simulink model "npc_controller"  (R2022a)
settings: Solver=FixedStepDiscrete  StartTime=0.0  StopTime=20  RelTol=1e-3  EnableMultiTasking=on
undefined symbols (not defined in the file): CAN_O_INT, CANA_BASE, Down, GPTRIP1SEL, GPTRIP2SEL, GPTRIP3SEL, Tsw, TZ1, TZ2, TZ3, Up, V2G_en
libraries: simulink x171, hdlsllib x90, c2802xlib x46, c2837xDlib x19, c280xlib x12, canmsglib x9, c2838xlib x8, idelinklib_common x5, c2806xlib x2, slpidlib x2, c28004xlib x2, c281xlib x2
(part 49 of 55)

== system npc_controller/CONTROL/STATE-MACHINE/CPU_CONTROL_100_A2_precharge_pfc_ok2/configGrid/FORCE_TZ/1P/LEG_A/System Outputs2 ==

== system npc_controller/CONTROL/STATE-MACHINE/CPU_CONTROL_100_A2_precharge_pfc_ok2/configGrid/FORCE_TZ/1P/LEG_B/System Outputs2 ==

== system npc_controller/CONTROL/STATE-MACHINE/CPU_CONTROL_100_A2_precharge_pfc_ok2/configGrid/FORCE_TZ/1P/LEG_C/System Outputs2 ==

== system npc_controller/CONTROL/STATE-MACHINE/CPU_CONTROL_100_A2_precharge_pfc_ok2/updatePll3p/PLL/SRF_PLL/Integrator/Accumulation ==
  In1 : Inport  OutDataTypeStr=single
  Action Port : ActionPort
  Out : Outport  OutDataTypeStr=single
  wires:
  In1/1 -> Out/1

== system npc_controller/CONTROL/STATE-MACHINE/CPU_CONTROL_100_A2_precharge_pfc_ok2/updatePll3p/PLL/SRF_PLL/Integrator/Reset Integrator ==
  Action Port : ActionPort
  Constant1 : Constant  Value=0  OutDataTypeStr=single
  Out : Outport
  wires:
  Constant1/1 -> Out/1

== system npc_controller/CONTROL/STATE-MACHINE/CPU_CONTROL_100_inv/configGrid/FORCE_TZ/1P/ALL_LEGS/System Outputs2 ==

== system npc_controller/CONTROL/STATE-MACHINE/CPU_CONTROL_100_inv/configGrid/FORCE_TZ/1P/LEG_A/System Outputs2 ==

== system npc_controller/CONTROL/STATE-MACHINE/CPU_CONTROL_100_inv/configGrid/FORCE_TZ/1P/LEG_B/System Outputs2 ==

== system npc_controller/CONTROL/STATE-MACHINE/CPU_CONTROL_100_inv/configGrid/FORCE_TZ/1P/LEG_C/System Outputs2 ==

== system npc_controller/CONTROL/STATE-MACHINE/CPU_CONTROL_100_inv/updatePll3p/PLL/SRF_PLL/Integrator/Accumulation ==
  In1 : Inport  OutDataTypeStr=single
  Action Port : ActionPort
  Out : Outport  OutDataTypeStr=single
  wires:
  In1/1 -> Out/1

== system npc_controller/CONTROL/STATE-MACHINE/CPU_CONTROL_100_inv/updatePll3p/PLL/SRF_PLL/Integrator/Reset Integrator ==
  Action Port : ActionPort
  Constant1 : Constant  Value=0  OutDataTypeStr=single
  Out : Outport
  wires:
  Constant1/1 -> Out/1

== system npc_controller/CONTROL/STATE-MACHINE/CPU_CONTROL_100_inv/updateSequencePhA/pol_vxn1/neg/SR OFF/System Outputs1 ==

== system npc_controller/CONTROL/STATE-MACHINE/CPU_CONTROL_100_inv/updateSequencePhA/pol_vxn1/neg/SR OFF/System Outputs2 ==

== system npc_controller/CONTROL/STATE-MACHINE/CPU_CONTROL_100_inv/updateSequencePhA/pol_vxn1/neg/SR ON/System Outputs1 ==

== system npc_controller/CONTROL/STATE-MACHINE/CPU_CONTROL_100_inv/updateSequencePhA/pol_vxn1/neg/SR ON/System Outputs2 ==

== system npc_controller/CONTROL/STATE-MACHINE/CPU_CONTROL_100_inv/updateSequencePhA/pol_vxn1/neg/SR ON1/System Outputs1 ==

== system npc_controller/CONTROL/STATE-MACHINE/CPU_CONTROL_100_inv/updateSequencePhA/pol_vxn1/neg/SR ON1/System Outputs2 ==

== system npc_controller/CONTROL/STATE-MACHINE/CPU_CONTROL_100_inv/updateSequencePhA/pol_vxn1/pos/S3_Blanking/System Outputs1 ==

== system npc_controller/CONTROL/STATE-MACHINE/CPU_CONTROL_100_inv/updateSequencePhA/pol_vxn1/pos/S3_Blanking/System Outputs2 ==

== system npc_controller/CONTROL/STATE-MACHINE/CPU_CONTROL_100_inv/updateSequencePhA/pol_vxn1/pos/SR Force to Low/System Outputs1 ==

== system npc_controller/CONTROL/STATE-MACHINE/CPU_CONTROL_100_inv/updateSequencePhA/pol_vxn1/pos/SR Force to Low/System Outputs2 ==

== system npc_controller/CONTROL/STATE-MACHINE/CPU_CONTROL_100_inv/updateSequencePhA/pol_vxn1/pos/SR ON/System Outputs1 ==

== system npc_controller/CONTROL/STATE-MACHINE/CPU_CONTROL_100_inv/updateSequencePhA/pol_vxn1/pos/SR ON/System Outputs2 ==

== system npc_controller/CONTROL/STATE-MACHINE/CPU_CONTROL_100_inv/updateSequencePhA1/pol_vxn1/neg/SR OFF/System Outputs1 ==

== system npc_controller/CONTROL/STATE-MACHINE/CPU_CONTROL_100_inv/updateSequencePhA1/pol_vxn1/neg/SR OFF/System Outputs2 ==

== system npc_controller/CONTROL/STATE-MACHINE/CPU_CONTROL_100_inv/updateSequencePhA1/pol_vxn1/neg/SR ON/System Outputs1 ==

== system npc_controller/CONTROL/STATE-MACHINE/CPU_CONTROL_100_inv/updateSequencePhA1/pol_vxn1/neg/SR ON/System Outputs2 ==

== system npc_controller/CONTROL/STATE-MACHINE/CPU_CONTROL_100_inv/updateSequencePhA1/pol_vxn1/pos/SR Force to Low/System Outputs1 ==

== system npc_controller/CONTROL/STATE-MACHINE/CPU_CONTROL_100_inv/updateSequencePhA1/pol_vxn1/pos/SR Force to Low/System Outputs2 ==

== system npc_controller/CONTROL/STATE-MACHINE/CPU_CONTROL_100_inv/updateSequencePhA1/pol_vxn1/pos/SR ON/System Outputs1 ==

== system npc_controller/CONTROL/STATE-MACHINE/CPU_CONTROL_100_inv/updateSequencePhA1/pol_vxn1/pos/SR ON/System Outputs2 ==

== system npc_controller/CONTROL/STATE-MACHINE/CPU_CONTROL_100_inv/updateSequencePhB/pol_vxn1/neg/SR OFF/System Outputs2 ==

== system npc_controller/CONTROL/STATE-MACHINE/CPU_CONTROL_100_inv/updateSequencePhB/pol_vxn1/neg/SR ON/System Outputs1 ==

== system npc_controller/CONTROL/STATE-MACHINE/CPU_CONTROL_100_inv/updateSequencePhB/pol_vxn1/neg/SR ON1/System Outputs1 ==

== system npc_controller/CONTROL/STATE-MACHINE/CPU_CONTROL_100_inv/updateSequencePhB/pol_vxn1/pos/SR Force to Low/System Outputs2 ==

== system npc_controller/CONTROL/STATE-MACHINE/CPU_CONTROL_100_inv/updateSequencePhB/pol_vxn1/pos/SR ON/System Outputs1 ==

== system npc_controller/CONTROL/STATE-MACHINE/CPU_CONTROL_100_inv/updateSequencePhB/pol_vxn1/pos/SR ON1/System Outputs1 ==

== system npc_controller/CONTROL/STATE-MACHINE/CPU_CONTROL_100_inv/updateSequencePhB1/pol_vxn1/neg/SR OFF/System Outputs2 ==

== system npc_controller/CONTROL/STATE-MACHINE/CPU_CONTROL_100_inv/updateSequencePhB1/pol_vxn1/neg/SR ON/System Outputs1 ==

== system npc_controller/CONTROL/STATE-MACHINE/CPU_CONTROL_100_inv/updateSequencePhB1/pol_vxn1/pos/SR Force to Low/System Outputs2 ==

== system npc_controller/CONTROL/STATE-MACHINE/CPU_CONTROL_100_inv/updateSequencePhB1/pol_vxn1/pos/SR ON/System Outputs1 ==

== system npc_controller/CONTROL/STATE-MACHINE/CPU_CONTROL_100_inv/updateSequencePhC/pol_vxn1/neg/S2_Blanking/System Outputs1 ==

== system npc_controller/CONTROL/STATE-MACHINE/CPU_CONTROL_100_inv/updateSequencePhC/pol_vxn1/neg/SR OFF/System Outputs1 ==

== system npc_controller/CONTROL/STATE-MACHINE/CPU_CONTROL_100_inv/updateSequencePhC/pol_vxn1/neg/SR ON/System Outputs1 ==

== system npc_controller/CONTROL/STATE-MACHINE/CPU_CONTROL_100_inv/updateSequencePhC/pol_vxn1/pos/S3_Blanking/System Outputs1 ==

== system npc_controller/CONTROL/STATE-MACHINE/CPU_CONTROL_100_inv/updateSequencePhC/pol_vxn1/pos/SR Force to Low/System Outputs2 ==

== system npc_controller/CONTROL/STATE-MACHINE/CPU_CONTROL_100_inv/updateSequencePhC/pol_vxn1/pos/SR ON/System Outputs1 ==

== system npc_controller/CONTROL/STATE-MACHINE/CPU_CONTROL_100_inv/updateSequencePhC1/pol_vxn1/neg/SR OFF/System Outputs1 ==

== system npc_controller/CONTROL/STATE-MACHINE/CPU_CONTROL_100_inv/updateSequencePhC1/pol_vxn1/neg/SR ON/System Outputs1 ==

== system npc_controller/CONTROL/STATE-MACHINE/CPU_CONTROL_100_inv/updateSequencePhC1/pol_vxn1/pos/SR Force to Low/System Outputs2 ==

== system npc_controller/CONTROL/STATE-MACHINE/CPU_CONTROL_100_inv/updateSequencePhC1/pol_vxn1/pos/SR ON/System Outputs1 ==

== system npc_controller/CONTROL/STATE-MACHINE/CPU_CONTROL_200_A2_precharge_pfc_ok2/configGrid/FORCE_TZ/1P/ALL_LEGS/System Outputs2 ==

== system npc_controller/CONTROL/STATE-MACHINE/CPU_CONTROL_200_A2_precharge_pfc_ok2/configGrid/FORCE_TZ/1P/LEG_A/System Outputs2 ==

== system npc_controller/CONTROL/STATE-MACHINE/CPU_CONTROL_200_A2_precharge_pfc_ok2/configGrid/FORCE_TZ/1P/LEG_B/System Outputs2 ==

== system npc_controller/CONTROL/STATE-MACHINE/CPU_CONTROL_200_A2_precharge_pfc_ok2/configGrid/FORCE_TZ/1P/LEG_C/System Outputs2 ==

== system npc_controller/CONTROL/STATE-MACHINE/CPU_CONTROL_200_A2_precharge_pfc_ok2/updatePll3p/PLL/SRF_PLL/Integrator/Accumulation ==
  In1 : Inport  OutDataTypeStr=single
  Action Port : ActionPort
  Out : Outport  OutDataTypeStr=single
  wires:
  In1/1 -> Out/1

== system npc_controller/CONTROL/STATE-MACHINE/CPU_CONTROL_200_A2_precharge_pfc_ok2/updatePll3p/PLL/SRF_PLL/Integrator/Reset Integrator ==
  Action Port : ActionPort
  Constant1 : Constant  Value=0  OutDataTypeStr=single
  Out : Outport
  wires:
  Constant1/1 -> Out/1

== system npc_controller/CONTROL/STATE-MACHINE/CPU_CONTROL_200_A2_precharge_pfc_ok2_OL SS/configGrid/FORCE_TZ/1P/ALL_LEGS/System Outputs2 ==

== system npc_controller/CONTROL/STATE-MACHINE/CPU_CONTROL_200_A2_precharge_pfc_ok2_OL SS/configGrid/FORCE_TZ/1P/LEG_A/System Outputs2 ==

== system npc_controller/CONTROL/STATE-MACHINE/CPU_CONTROL_200_A2_precharge_pfc_ok2_OL SS/configGrid/FORCE_TZ/1P/LEG_B/System Outputs2 ==

== system npc_controller/CONTROL/STATE-MACHINE/CPU_CONTROL_200_A2_precharge_pfc_ok2_OL SS/configGrid/FORCE_TZ/1P/LEG_C/System Outputs2 ==

== system npc_controller/CONTROL/STATE-MACHINE/CPU_CONTROL_200_A2_precharge_pfc_ok2_OL SS/updatePll3p/PLL/SRF_PLL/Integrator/Accumulation ==
  In1 : Inport  OutDataTypeStr=single
  Action Port : ActionPort
  Out : Outport  OutDataTypeStr=single
  wires:
  In1/1 -> Out/1

== system npc_controller/CONTROL/STATE-MACHINE/CPU_CONTROL_200_A2_precharge_pfc_ok2_OL SS/updatePll3p/PLL/SRF_PLL/Integrator/Reset Integrator ==
  Action Port : ActionPort
  Constant1 : Constant  Value=0  OutDataTypeStr=single
  Out : Outport
  wires:
  Constant1/1 -> Out/1

== system npc_controller/CONTROL/STATE-MACHINE/CPU_CONTROL_200_Vpk/configGrid/FORCE_TZ/1P/ALL_LEGS/System Outputs2 ==

== system npc_controller/CONTROL/STATE-MACHINE/CPU_CONTROL_200_Vpk/configGrid/FORCE_TZ/1P/LEG_A/System Outputs2 ==

== system npc_controller/CONTROL/STATE-MACHINE/CPU_CONTROL_200_Vpk/configGrid/FORCE_TZ/1P/LEG_B/System Outputs2 ==

== system npc_controller/CONTROL/STATE-MACHINE/CPU_CONTROL_200_Vpk/configGrid/FORCE_TZ/1P/LEG_C/System Outputs2 ==

== system npc_controller/CONTROL/STATE-MACHINE/CPU_CONTROL_200_Vpk/updatePll3p/PLL/SRF_PLL/Integrator/Accumulation ==
  In1 : Inport  OutDataTypeStr=single
  Action Port : ActionPort
  Out : Outport  OutDataTypeStr=single
  wires:
  In1/1 -> Out/1

== system npc_controller/CONTROL/STATE-MACHINE/CPU_CONTROL_200_Vpk/updatePll3p/PLL/SRF_PLL/Integrator/Reset Integrator ==
  Action Port : ActionPort
  Constant1 : Constant  Value=0  OutDataTypeStr=single
  Out : Outport
  wires:
  Constant1/1 -> Out/1

== system npc_controller/CONTROL/STATE-MACHINE/CPU_CONTROL_200_inv/configGrid/FORCE_TZ/1P/ALL_LEGS/System Outputs2 ==

== system npc_controller/CONTROL/STATE-MACHINE/CPU_CONTROL_200_inv/configGrid/FORCE_TZ/1P/LEG_A/System Outputs2 ==

== system npc_controller/CONTROL/STATE-MACHINE/CPU_CONTROL_200_inv/configGrid/FORCE_TZ/1P/LEG_B/System Outputs2 ==

== system npc_controller/CONTROL/STATE-MACHINE/CPU_CONTROL_200_inv/configGrid/FORCE_TZ/1P/LEG_C/System Outputs2 ==

== system npc_controller/CONTROL/STATE-MACHINE/CPU_CONTROL_200_inv/updatePll3p/PLL/SRF_PLL/Integrator/Accumulation ==
  In1 : Inport  OutDataTypeStr=single
  Action Port : ActionPort
  Out : Outport  OutDataTypeStr=single
  wires:
  In1/1 -> Out/1

== system npc_controller/CONTROL/STATE-MACHINE/CPU_CONTROL_200_inv/updatePll3p/PLL/SRF_PLL/Integrator/Reset Integrator ==
  Action Port : ActionPort
  Constant1 : Constant  Value=0  OutDataTypeStr=single
  Out : Outport
  wires:
  Constant1/1 -> Out/1

== system npc_controller/CONTROL/STATE-MACHINE/CPU_CONTROL_200_inv/updateSequencePhA/pol_vxn1/neg/SR OFF/System Outputs1 ==

== system npc_controller/CONTROL/STATE-MACHINE/CPU_CONTROL_200_inv/updateSequencePhA/pol_vxn1/neg/SR OFF/System Outputs2 ==

== system npc_controller/CONTROL/STATE-MACHINE/CPU_CONTROL_200_inv/updateSequencePhA/pol_vxn1/neg/SR ON/System Outputs1 ==

== system npc_controller/CONTROL/STATE-MACHINE/CPU_CONTROL_200_inv/updateSequencePhA/pol_vxn1/neg/SR ON/System Outputs2 ==

== system npc_controller/CONTROL/STATE-MACHINE/CPU_CONTROL_200_inv/updateSequencePhA/pol_vxn1/neg/SR ON1/System Outputs1 ==

== system npc_controller/CONTROL/STATE-MACHINE/CPU_CONTROL_200_inv/updateSequencePhA/pol_vxn1/neg/SR ON1/System Outputs2 ==

== system npc_controller/CONTROL/STATE-MACHINE/CPU_CONTROL_200_inv/updateSequencePhA/pol_vxn1/pos/S3_Blanking/System Outputs1 ==

== system npc_controller/CONTROL/STATE-MACHINE/CPU_CONTROL_200_inv/updateSequencePhA/pol_vxn1/pos/S3_Blanking/System Outputs2 ==

== system npc_controller/CONTROL/STATE-MACHINE/CPU_CONTROL_200_inv/updateSequencePhA/pol_vxn1/pos/SR Force to Low/System Outputs1 ==

== system npc_controller/CONTROL/STATE-MACHINE/CPU_CONTROL_200_inv/updateSequencePhA/pol_vxn1/pos/SR Force to Low/System Outputs2 ==

== system npc_controller/CONTROL/STATE-MACHINE/CPU_CONTROL_200_inv/updateSequencePhA/pol_vxn1/pos/SR ON/System Outputs1 ==

== system npc_controller/CONTROL/STATE-MACHINE/CPU_CONTROL_200_inv/updateSequencePhA/pol_vxn1/pos/SR ON/System Outputs2 ==

== system npc_controller/CONTROL/STATE-MACHINE/CPU_CONTROL_200_inv/updateSequencePhA1/pol_vxn1/neg/SR OFF/System Outputs1 ==

== system npc_controller/CONTROL/STATE-MACHINE/CPU_CONTROL_200_inv/updateSequencePhA1/pol_vxn1/neg/SR OFF/System Outputs2 ==

== system npc_controller/CONTROL/STATE-MACHINE/CPU_CONTROL_200_inv/updateSequencePhA1/pol_vxn1/neg/SR ON/System Outputs1 ==

== system npc_controller/CONTROL/STATE-MACHINE/CPU_CONTROL_200_inv/updateSequencePhA1/pol_vxn1/neg/SR ON/System Outputs2 ==

== system npc_controller/CONTROL/STATE-MACHINE/CPU_CONTROL_200_inv/updateSequencePhA1/pol_vxn1/pos/SR Force to Low/System Outputs1 ==

== system npc_controller/CONTROL/STATE-MACHINE/CPU_CONTROL_200_inv/updateSequencePhA1/pol_vxn1/pos/SR Force to Low/System Outputs2 ==

== system npc_controller/CONTROL/STATE-MACHINE/CPU_CONTROL_200_inv/updateSequencePhA1/pol_vxn1/pos/SR ON/System Outputs1 ==

== system npc_controller/CONTROL/STATE-MACHINE/CPU_CONTROL_200_inv/updateSequencePhA1/pol_vxn1/pos/SR ON/System Outputs2 ==

== system npc_controller/CONTROL/STATE-MACHINE/CPU_CONTROL_200_inv/updateSequencePhB/pol_vxn1/neg/SR OFF/System Outputs2 ==

== system npc_controller/CONTROL/STATE-MACHINE/CPU_CONTROL_200_inv/updateSequencePhB/pol_vxn1/neg/SR ON/System Outputs1 ==

== system npc_controller/CONTROL/STATE-MACHINE/CPU_CONTROL_200_inv/updateSequencePhB/pol_vxn1/neg/SR ON1/System Outputs1 ==

== system npc_controller/CONTROL/STATE-MACHINE/CPU_CONTROL_200_inv/updateSequencePhB/pol_vxn1/pos/SR Force to Low/System Outputs2 ==

== system npc_controller/CONTROL/STATE-MACHINE/CPU_CONTROL_200_inv/updateSequencePhB/pol_vxn1/pos/SR ON/System Outputs1 ==

== system npc_controller/CONTROL/STATE-MACHINE/CPU_CONTROL_200_inv/updateSequencePhB/pol_vxn1/pos/SR ON1/System Outputs1 ==

== system npc_controller/CONTROL/STATE-MACHINE/CPU_CONTROL_200_inv/updateSequencePhB1/pol_vxn1/neg/SR OFF/System Outputs2 ==

== system npc_controller/CONTROL/STATE-MACHINE/CPU_CONTROL_200_inv/updateSequencePhB1/pol_vxn1/neg/SR ON/System Outputs1 ==

== system npc_controller/CONTROL/STATE-MACHINE/CPU_CONTROL_200_inv/updateSequencePhB1/pol_vxn1/pos/SR Force to Low/System Outputs2 ==

== system npc_controller/CONTROL/STATE-MACHINE/CPU_CONTROL_200_inv/updateSequencePhB1/pol_vxn1/pos/SR ON/System Outputs1 ==

== system npc_controller/CONTROL/STATE-MACHINE/CPU_CONTROL_200_inv/updateSequencePhC/pol_vxn1/neg/S2_Blanking/System Outputs1 ==

== system npc_controller/CONTROL/STATE-MACHINE/CPU_CONTROL_200_inv/updateSequencePhC/pol_vxn1/neg/SR OFF/System Outputs1 ==

== system npc_controller/CONTROL/STATE-MACHINE/CPU_CONTROL_200_inv/updateSequencePhC/pol_vxn1/neg/SR ON/System Outputs1 ==

== system npc_controller/CONTROL/STATE-MACHINE/CPU_CONTROL_200_inv/updateSequencePhC/pol_vxn1/pos/S3_Blanking/System Outputs1 ==

== system npc_controller/CONTROL/STATE-MACHINE/CPU_CONTROL_200_inv/updateSequencePhC/pol_vxn1/pos/SR Force to Low/System Outputs2 ==

== system npc_controller/CONTROL/STATE-MACHINE/CPU_CONTROL_200_inv/updateSequencePhC/pol_vxn1/pos/SR ON/System Outputs1 ==

== system npc_controller/CONTROL/STATE-MACHINE/CPU_CONTROL_200_inv/updateSequencePhC1/pol_vxn1/neg/SR OFF/System Outputs1 ==

== system npc_controller/CONTROL/STATE-MACHINE/CPU_CONTROL_200_inv/updateSequencePhC1/pol_vxn1/neg/SR ON/System Outputs1 ==

== system npc_controller/CONTROL/STATE-MACHINE/CPU_CONTROL_200_inv/updateSequencePhC1/pol_vxn1/pos/SR Force to Low/System Outputs2 ==

== system npc_controller/CONTROL/STATE-MACHINE/CPU_CONTROL_200_inv/updateSequencePhC1/pol_vxn1/pos/SR ON/System Outputs1 ==

== system npc_controller/CONTROL/STATE-MACHINE/CPU_CONTROL_400/configGrid/FORCE_TZ/1P/ALL_LEGS/System Outputs2 ==

== system npc_controller/CONTROL/STATE-MACHINE/CPU_CONTROL_400/configGrid/FORCE_TZ/1P/LEG_A/System Outputs2 ==

== system npc_controller/CONTROL/STATE-MACHINE/CPU_CONTROL_400/configGrid/FORCE_TZ/1P/LEG_B/System Outputs2 ==

== system npc_controller/CONTROL/STATE-MACHINE/CPU_CONTROL_400/configGrid/FORCE_TZ/1P/LEG_C/System Outputs2 ==

== system npc_controller/CONTROL/STATE-MACHINE/CPU_CONTROL_400/updatePll3p/PLL/SRF_PLL/Integrator/Accumulation ==
  In1 : Inport  OutDataTypeStr=single
  Action Port : ActionPort
  Out : Outport  OutDataTypeStr=single
  wires:
  In1/1 -> Out/1

== system npc_controller/CONTROL/STATE-MACHINE/CPU_CONTROL_400/updatePll3p/PLL/SRF_PLL/Integrator/Reset Integrator ==
  Action Port : ActionPort
  Constant1 : Constant  Value=0  OutDataTypeStr=single
  Out : Outport
  wires:
  Constant1/1 -> Out/1

== system npc_controller/CONTROL/STATE-MACHINE/CPU_CONTROL_400_A2_precharge_pfc_ok2_OL SS/configGrid/FORCE_TZ/1P/ALL_LEGS/System Outputs2 ==

== system npc_controller/CONTROL/STATE-MACHINE/CPU_CONTROL_400_A2_precharge_pfc_ok2_OL SS/configGrid/FORCE_TZ/1P/LEG_A/System Outputs2 ==

== system npc_controller/CONTROL/STATE-MACHINE/CPU_CONTROL_400_A2_precharge_pfc_ok2_OL SS/configGrid/FORCE_TZ/1P/LEG_B/System Outputs2 ==

== system npc_controller/CONTROL/STATE-MACHINE/CPU_CONTROL_400_A2_precharge_pfc_ok2_OL SS/configGrid/FORCE_TZ/1P/LEG_C/System Outputs2 ==

== system npc_controller/CONTROL/STATE-MACHINE/CPU_CONTROL_400_A2_precharge_pfc_ok2_OL SS/updatePll3p/PLL/SRF_PLL/Integrator/Accumulation ==
  In1 : Inport  OutDataTypeStr=single
  Action Port : ActionPort
  Out : Outport  OutDataTypeStr=single
  wires:
  In1/1 -> Out/1

== system npc_controller/CONTROL/STATE-MACHINE/CPU_CONTROL_400_A2_precharge_pfc_ok2_OL SS/updatePll3p/PLL/SRF_PLL/Integrator/Reset Integrator ==
  Action Port : ActionPort
  Constant1 : Constant  Value=0  OutDataTypeStr=single
  Out : Outport
  wires:
  Constant1/1 -> Out/1

== system npc_controller/CONTROL/STATE-MACHINE/CPU_CONTROL_400_inv/configGrid/FORCE_TZ/1P/ALL_LEGS/System Outputs2 ==

== system npc_controller/CONTROL/STATE-MACHINE/CPU_CONTROL_400_inv/configGrid/FORCE_TZ/1P/LEG_A/System Outputs2 ==

== system npc_controller/CONTROL/STATE-MACHINE/CPU_CONTROL_400_inv/configGrid/FORCE_TZ/1P/LEG_B/System Outputs2 ==

== system npc_controller/CONTROL/STATE-MACHINE/CPU_CONTROL_400_inv/configGrid/FORCE_TZ/1P/LEG_C/System Outputs2 ==

== system npc_controller/CONTROL/STATE-MACHINE/CPU_CONTROL_400_inv/updatePll3p/PLL/SRF_PLL/Integrator/Accumulation ==
  In1 : Inport  OutDataTypeStr=single
  Action Port : ActionPort
  Out : Outport  OutDataTypeStr=single
  wires:
  In1/1 -> Out/1

== system npc_controller/CONTROL/STATE-MACHINE/CPU_CONTROL_400_inv/updatePll3p/PLL/SRF_PLL/Integrator/Reset Integrator ==
  Action Port : ActionPort
  Constant1 : Constant  Value=0  OutDataTypeStr=single
  Out : Outport
  wires:
  Constant1/1 -> Out/1

== system npc_controller/CONTROL/STATE-MACHINE/CPU_CONTROL_400_inv/updateSequencePhA/pol_vxn1/neg/SR OFF/System Outputs1 ==

== system npc_controller/CONTROL/STATE-MACHINE/CPU_CONTROL_400_inv/updateSequencePhA/pol_vxn1/neg/SR OFF/System Outputs2 ==

== system npc_controller/CONTROL/STATE-MACHINE/CPU_CONTROL_400_inv/updateSequencePhA/pol_vxn1/neg/SR ON/System Outputs1 ==

== system npc_controller/CONTROL/STATE-MACHINE/CPU_CONTROL_400_inv/updateSequencePhA/pol_vxn1/neg/SR ON/System Outputs2 ==

== system npc_controller/CONTROL/STATE-MACHINE/CPU_CONTROL_400_inv/updateSequencePhA/pol_vxn1/neg/SR ON1/System Outputs1 ==

== system npc_controller/CONTROL/STATE-MACHINE/CPU_CONTROL_400_inv/updateSequencePhA/pol_vxn1/neg/SR ON1/System Outputs2 ==

== system npc_controller/CONTROL/STATE-MACHINE/CPU_CONTROL_400_inv/updateSequencePhA/pol_vxn1/pos/S3_Blanking/System Outputs1 ==

== system npc_controller/CONTROL/STATE-MACHINE/CPU_CONTROL_400_inv/updateSequencePhA/pol_vxn1/pos/S3_Blanking/System Outputs2 ==

== system npc_controller/CONTROL/STATE-MACHINE/CPU_CONTROL_400_inv/updateSequencePhA/pol_vxn1/pos/SR Force to Low/System Outputs1 ==

== system npc_controller/CONTROL/STATE-MACHINE/CPU_CONTROL_400_inv/updateSequencePhA/pol_vxn1/pos/SR Force to Low/System Outputs2 ==

== system npc_controller/CONTROL/STATE-MACHINE/CPU_CONTROL_400_inv/updateSequencePhA/pol_vxn1/pos/SR ON/System Outputs1 ==

== system npc_controller/CONTROL/STATE-MACHINE/CPU_CONTROL_400_inv/updateSequencePhA/pol_vxn1/pos/SR ON/System Outputs2 ==

== system npc_controller/CONTROL/STATE-MACHINE/CPU_CONTROL_400_inv/updateSequencePhA1/pol_vxn1/neg/SR OFF/System Outputs1 ==

== system npc_controller/CONTROL/STATE-MACHINE/CPU_CONTROL_400_inv/updateSequencePhA1/pol_vxn1/neg/SR OFF/System Outputs2 ==

== system npc_controller/CONTROL/STATE-MACHINE/CPU_CONTROL_400_inv/updateSequencePhA1/pol_vxn1/neg/SR ON/System Outputs1 ==

== system npc_controller/CONTROL/STATE-MACHINE/CPU_CONTROL_400_inv/updateSequencePhA1/pol_vxn1/neg/SR ON/System Outputs2 ==

== system npc_controller/CONTROL/STATE-MACHINE/CPU_CONTROL_400_inv/updateSequencePhA1/pol_vxn1/pos/SR Force to Low/System Outputs1 ==

== system npc_controller/CONTROL/STATE-MACHINE/CPU_CONTROL_400_inv/updateSequencePhA1/pol_vxn1/pos/SR Force to Low/System Outputs2 ==

== system npc_controller/CONTROL/STATE-MACHINE/CPU_CONTROL_400_inv/updateSequencePhA1/pol_vxn1/pos/SR ON/System Outputs1 ==

== system npc_controller/CONTROL/STATE-MACHINE/CPU_CONTROL_400_inv/updateSequencePhA1/pol_vxn1/pos/SR ON/System Outputs2 ==

== system npc_controller/CONTROL/STATE-MACHINE/CPU_CONTROL_400_inv/updateSequencePhB/pol_vxn1/neg/SR OFF/System Outputs2 ==

== system npc_controller/CONTROL/STATE-MACHINE/CPU_CONTROL_400_inv/updateSequencePhB/pol_vxn1/neg/SR ON/System Outputs1 ==

== system npc_controller/CONTROL/STATE-MACHINE/CPU_CONTROL_400_inv/updateSequencePhB/pol_vxn1/neg/SR ON1/System Outputs1 ==

== system npc_controller/CONTROL/STATE-MACHINE/CPU_CONTROL_400_inv/updateSequencePhB/pol_vxn1/pos/SR Force to Low/System Outputs2 ==

== system npc_controller/CONTROL/STATE-MACHINE/CPU_CONTROL_400_inv/updateSequencePhB/pol_vxn1/pos/SR ON/System Outputs1 ==

== system npc_controller/CONTROL/STATE-MACHINE/CPU_CONTROL_400_inv/updateSequencePhB/pol_vxn1/pos/SR ON1/System Outputs1 ==

== system npc_controller/CONTROL/STATE-MACHINE/CPU_CONTROL_400_inv/updateSequencePhB1/pol_vxn1/neg/SR OFF/System Outputs2 ==

== system npc_controller/CONTROL/STATE-MACHINE/CPU_CONTROL_400_inv/updateSequencePhB1/pol_vxn1/neg/SR ON/System Outputs1 ==

== system npc_controller/CONTROL/STATE-MACHINE/CPU_CONTROL_400_inv/updateSequencePhB1/pol_vxn1/pos/SR Force to Low/System Outputs2 ==

== system npc_controller/CONTROL/STATE-MACHINE/CPU_CONTROL_400_inv/updateSequencePhB1/pol_vxn1/pos/SR ON/System Outputs1 ==

== system npc_controller/CONTROL/STATE-MACHINE/CPU_CONTROL_400_inv/updateSequencePhC/pol_vxn1/neg/S2_Blanking/System Outputs1 ==

== system npc_controller/CONTROL/STATE-MACHINE/CPU_CONTROL_400_inv/updateSequencePhC/pol_vxn1/neg/SR OFF/System Outputs1 ==

== system npc_controller/CONTROL/STATE-MACHINE/CPU_CONTROL_400_inv/updateSequencePhC/pol_vxn1/neg/SR ON/System Outputs1 ==

== system npc_controller/CONTROL/STATE-MACHINE/CPU_CONTROL_400_inv/updateSequencePhC/pol_vxn1/pos/S3_Blanking/System Outputs1 ==

== system npc_controller/CONTROL/STATE-MACHINE/CPU_CONTROL_400_inv/updateSequencePhC/pol_vxn1/pos/SR Force to Low/System Outputs2 ==

== system npc_controller/CONTROL/STATE-MACHINE/CPU_CONTROL_400_inv/updateSequencePhC/pol_vxn1/pos/SR ON/System Outputs1 ==

== system npc_controller/CONTROL/STATE-MACHINE/CPU_CONTROL_400_inv/updateSequencePhC1/pol_vxn1/neg/SR OFF/System Outputs1 ==

== system npc_controller/CONTROL/STATE-MACHINE/CPU_CONTROL_400_inv/updateSequencePhC1/pol_vxn1/neg/SR ON/System Outputs1 ==

== system npc_controller/CONTROL/STATE-MACHINE/CPU_CONTROL_400_inv/updateSequencePhC1/pol_vxn1/pos/SR Force to Low/System Outputs2 ==

== system npc_controller/CONTROL/STATE-MACHINE/CPU_CONTROL_400_inv/updateSequencePhC1/pol_vxn1/pos/SR ON/System Outputs1 ==

== system npc_controller/CONTROL/STATE-MACHINE/CPU_CONTROL_750_A2_precharge_pfc_ok1/configGrid/FORCE_TZ/1P/ALL_LEGS/System Outputs2 ==

== system npc_controller/CONTROL/STATE-MACHINE/CPU_CONTROL_750_A2_precharge_pfc_ok1/configGrid/FORCE_TZ/1P/LEG_A/System Outputs2 ==

== system npc_controller/CONTROL/STATE-MACHINE/CPU_CONTROL_750_A2_precharge_pfc_ok1/configGrid/FORCE_TZ/1P/LEG_B/System Outputs2 ==

== system npc_controller/CONTROL/STATE-MACHINE/CPU_CONTROL_750_A2_precharge_pfc_ok1/configGrid/FORCE_TZ/1P/LEG_C/System Outputs2 ==

== system npc_controller/CONTROL/STATE-MACHINE/CPU_CONTROL_750_A2_precharge_pfc_ok1/updatePll3p/PLL/SRF_PLL/Integrator/Accumulation ==
  In1 : Inport  OutDataTypeStr=single
  Action Port : ActionPort
  Out : Outport  OutDataTypeStr=single
  wires:
  In1/1 -> Out/1

== system npc_controller/CONTROL/STATE-MACHINE/CPU_CONTROL_750_A2_precharge_pfc_ok1/updatePll3p/PLL/SRF_PLL/Integrator/Reset Integrator ==
  Action Port : ActionPort
  Constant1 : Constant  Value=0  OutDataTypeStr=single
  Out : Outport
  wires:
  Constant1/1 -> Out/1

== system npc_controller/CONTROL/STATE-MACHINE/CPU_CONTROL_750_A2_precharge_pfc_ok2_OL SS1/configGrid/FORCE_TZ/1P/ALL_LEGS/System Outputs2 ==

== system npc_controller/CONTROL/STATE-MACHINE/CPU_CONTROL_750_A2_precharge_pfc_ok2_OL SS1/configGrid/FORCE_TZ/1P/LEG_A/System Outputs2 ==

== system npc_controller/CONTROL/STATE-MACHINE/CPU_CONTROL_750_A2_precharge_pfc_ok2_OL SS1/configGrid/FORCE_TZ/1P/LEG_B/System Outputs2 ==

== system npc_controller/CONTROL/STATE-MACHINE/CPU_CONTROL_750_A2_precharge_pfc_ok2_OL SS1/configGrid/FORCE_TZ/1P/LEG_C/System Outputs2 ==

== system npc_controller/CONTROL/STATE-MACHINE/CPU_CONTROL_750_A2_precharge_pfc_ok2_OL SS1/updatePll3p/PLL/SRF_PLL/Integrator/Accumulation ==
  In1 : Inport  OutDataTypeStr=single
  Action Port : ActionPort
  Out : Outport  OutDataTypeStr=single
  wires:
  In1/1 -> Out/1

== system npc_controller/CONTROL/STATE-MACHINE/CPU_CONTROL_750_A2_precharge_pfc_ok2_OL SS1/updatePll3p/PLL/SRF_PLL/Integrator/Reset Integrator ==
  Action Port : ActionPort
  Constant1 : Constant  Value=0  OutDataTypeStr=single
  Out : Outport
  wires:
  Constant1/1 -> Out/1

== system npc_controller/CONTROL/STATE-MACHINE/CPU_CONTROL_750_Vpk/configGrid/FORCE_TZ/1P/ALL_LEGS/System Outputs2 ==

== system npc_controller/CONTROL/STATE-MACHINE/CPU_CONTROL_750_Vpk/configGrid/FORCE_TZ/1P/LEG_A/System Outputs2 ==

== system npc_controller/CONTROL/STATE-MACHINE/CPU_CONTROL_750_Vpk/configGrid/FORCE_TZ/1P/LEG_B/System Outputs2 ==

== system npc_controller/CONTROL/STATE-MACHINE/CPU_CONTROL_750_Vpk/configGrid/FORCE_TZ/1P/LEG_C/System Outputs2 ==

== system npc_controller/CONTROL/STATE-MACHINE/CPU_CONTROL_750_Vpk/updatePll3p/PLL/SRF_PLL/Integrator/Accumulation ==
  In1 : Inport  OutDataTypeStr=single
  Action Port : ActionPort
  Out : Outport  OutDataTypeStr=single
  wires:
  In1/1 -> Out/1

== system npc_controller/CONTROL/STATE-MACHINE/CPU_CONTROL_750_Vpk/updatePll3p/PLL/SRF_PLL/Integrator/Reset Integrator ==
  Action Port : ActionPort
  Constant1 : Constant  Value=0  OutDataTypeStr=single
  Out : Outport
  wires:
  Constant1/1 -> Out/1

== system npc_controller/CONTROL/STATE-MACHINE/CPU_CONTROL_750_inv/configGrid/FORCE_TZ/1P/ALL_LEGS/System Outputs2 ==

== system npc_controller/CONTROL/STATE-MACHINE/CPU_CONTROL_750_inv/configGrid/FORCE_TZ/1P/LEG_A/System Outputs2 ==

== system npc_controller/CONTROL/STATE-MACHINE/CPU_CONTROL_750_inv/configGrid/FORCE_TZ/1P/LEG_B/System Outputs2 ==

== system npc_controller/CONTROL/STATE-MACHINE/CPU_CONTROL_750_inv/configGrid/FORCE_TZ/1P/LEG_C/System Outputs2 ==

== system npc_controller/CONTROL/STATE-MACHINE/CPU_CONTROL_750_inv/updatePll3p/PLL/SRF_PLL/Integrator/Accumulation ==
  In1 : Inport  OutDataTypeStr=single
  Action Port : ActionPort
  Out : Outport  OutDataTypeStr=single
  wires:
  In1/1 -> Out/1

== system npc_controller/CONTROL/STATE-MACHINE/CPU_CONTROL_750_inv/updatePll3p/PLL/SRF_PLL/Integrator/Reset Integrator ==
  Action Port : ActionPort
  Constant1 : Constant  Value=0  OutDataTypeStr=single
  Out : Outport
  wires:
  Constant1/1 -> Out/1

== system npc_controller/CONTROL/STATE-MACHINE/CPU_CONTROL_750_inv/updateSequencePhA/pol_vxn1/neg/SR OFF/System Outputs1 ==

== system npc_controller/CONTROL/STATE-MACHINE/CPU_CONTROL_750_inv/updateSequencePhA/pol_vxn1/neg/SR OFF/System Outputs2 ==

== system npc_controller/CONTROL/STATE-MACHINE/CPU_CONTROL_750_inv/updateSequencePhA/pol_vxn1/neg/SR ON/System Outputs1 ==

== system npc_controller/CONTROL/STATE-MACHINE/CPU_CONTROL_750_inv/updateSequencePhA/pol_vxn1/neg/SR ON/System Outputs2 ==

== system npc_controller/CONTROL/STATE-MACHINE/CPU_CONTROL_750_inv/updateSequencePhA/pol_vxn1/neg/SR ON1/System Outputs1 ==

== system npc_controller/CONTROL/STATE-MACHINE/CPU_CONTROL_750_inv/updateSequencePhA/pol_vxn1/neg/SR ON1/System Outputs2 ==

== system npc_controller/CONTROL/STATE-MACHINE/CPU_CONTROL_750_inv/updateSequencePhA/pol_vxn1/pos/S3_Blanking/System Outputs1 ==

== system npc_controller/CONTROL/STATE-MACHINE/CPU_CONTROL_750_inv/updateSequencePhA/pol_vxn1/pos/S3_Blanking/System Outputs2 ==

== system npc_controller/CONTROL/STATE-MACHINE/CPU_CONTROL_750_inv/updateSequencePhA/pol_vxn1/pos/SR Force to Low/System Outputs1 ==

== system npc_controller/CONTROL/STATE-MACHINE/CPU_CONTROL_750_inv/updateSequencePhA/pol_vxn1/pos/SR Force to Low/System Outputs2 ==

== system npc_controller/CONTROL/STATE-MACHINE/CPU_CONTROL_750_inv/updateSequencePhA/pol_vxn1/pos/SR ON/System Outputs1 ==

== system npc_controller/CONTROL/STATE-MACHINE/CPU_CONTROL_750_inv/updateSequencePhA/pol_vxn1/pos/SR ON/System Outputs2 ==

== system npc_controller/CONTROL/STATE-MACHINE/CPU_CONTROL_750_inv/updateSequencePhA1/pol_vxn1/neg/SR OFF/System Outputs1 ==

== system npc_controller/CONTROL/STATE-MACHINE/CPU_CONTROL_750_inv/updateSequencePhA1/pol_vxn1/neg/SR OFF/System Outputs2 ==

== system npc_controller/CONTROL/STATE-MACHINE/CPU_CONTROL_750_inv/updateSequencePhA1/pol_vxn1/neg/SR ON/System Outputs1 ==

== system npc_controller/CONTROL/STATE-MACHINE/CPU_CONTROL_750_inv/updateSequencePhA1/pol_vxn1/neg/SR ON/System Outputs2 ==

== system npc_controller/CONTROL/STATE-MACHINE/CPU_CONTROL_750_inv/updateSequencePhA1/pol_vxn1/pos/SR Force to Low/System Outputs1 ==

== system npc_controller/CONTROL/STATE-MACHINE/CPU_CONTROL_750_inv/updateSequencePhA1/pol_vxn1/pos/SR Force to Low/System Outputs2 ==

== system npc_controller/CONTROL/STATE-MACHINE/CPU_CONTROL_750_inv/updateSequencePhA1/pol_vxn1/pos/SR ON/System Outputs1 ==

== system npc_controller/CONTROL/STATE-MACHINE/CPU_CONTROL_750_inv/updateSequencePhA1/pol_vxn1/pos/SR ON/System Outputs2 ==

== system npc_controller/CONTROL/STATE-MACHINE/CPU_CONTROL_750_inv/updateSequencePhB/pol_vxn1/neg/SR OFF/System Outputs2 ==

== system npc_controller/CONTROL/STATE-MACHINE/CPU_CONTROL_750_inv/updateSequencePhB/pol_vxn1/neg/SR ON/System Outputs1 ==

== system npc_controller/CONTROL/STATE-MACHINE/CPU_CONTROL_750_inv/updateSequencePhB/pol_vxn1/neg/SR ON1/System Outputs1 ==

== system npc_controller/CONTROL/STATE-MACHINE/CPU_CONTROL_750_inv/updateSequencePhB/pol_vxn1/pos/SR Force to Low/System Outputs2 ==

== system npc_controller/CONTROL/STATE-MACHINE/CPU_CONTROL_750_inv/updateSequencePhB/pol_vxn1/pos/SR ON/System Outputs1 ==

== system npc_controller/CONTROL/STATE-MACHINE/CPU_CONTROL_750_inv/updateSequencePhB/pol_vxn1/pos/SR ON1/System Outputs1 ==

== system npc_controller/CONTROL/STATE-MACHINE/CPU_CONTROL_750_inv/updateSequencePhB1/pol_vxn1/neg/SR OFF/System Outputs2 ==

== system npc_controller/CONTROL/STATE-MACHINE/CPU_CONTROL_750_inv/updateSequencePhB1/pol_vxn1/neg/SR ON/System Outputs1 ==

== system npc_controller/CONTROL/STATE-MACHINE/CPU_CONTROL_750_inv/updateSequencePhB1/pol_vxn1/pos/SR Force to Low/System Outputs2 ==

== system npc_controller/CONTROL/STATE-MACHINE/CPU_CONTROL_750_inv/updateSequencePhB1/pol_vxn1/pos/SR ON/System Outputs1 ==

== system npc_controller/CONTROL/STATE-MACHINE/CPU_CONTROL_750_inv/updateSequencePhC/pol_vxn1/neg/S2_Blanking/System Outputs1 ==

== system npc_controller/CONTROL/STATE-MACHINE/CPU_CONTROL_750_inv/updateSequencePhC/pol_vxn1/neg/SR OFF/System Outputs1 ==

== system npc_controller/CONTROL/STATE-MACHINE/CPU_CONTROL_750_inv/updateSequencePhC/pol_vxn1/neg/SR ON/System Outputs1 ==

== system npc_controller/CONTROL/STATE-MACHINE/CPU_CONTROL_750_inv/updateSequencePhC/pol_vxn1/pos/S3_Blanking/System Outputs1 ==

== system npc_controller/CONTROL/STATE-MACHINE/CPU_CONTROL_750_inv/updateSequencePhC/pol_vxn1/pos/SR Force to Low/System Outputs2 ==

== system npc_controller/CONTROL/STATE-MACHINE/CPU_CONTROL_750_inv/updateSequencePhC/pol_vxn1/pos/SR ON/System Outputs1 ==

== system npc_controller/CONTROL/STATE-MACHINE/CPU_CONTROL_750_inv/updateSequencePhC1/pol_vxn1/neg/SR OFF/System Outputs1 ==

== system npc_controller/CONTROL/STATE-MACHINE/CPU_CONTROL_750_inv/updateSequencePhC1/pol_vxn1/neg/SR ON/System Outputs1 ==

== system npc_controller/CONTROL/STATE-MACHINE/CPU_CONTROL_750_inv/updateSequencePhC1/pol_vxn1/pos/SR Force to Low/System Outputs2 ==

== system npc_controller/CONTROL/STATE-MACHINE/CPU_CONTROL_750_inv/updateSequencePhC1/pol_vxn1/pos/SR ON/System Outputs1 ==

== system npc_controller/CONTROL/STATE-MACHINE/CPU_CONTROL_750_precharge_pfc_ok2/configGrid/FORCE_TZ/1P/ALL_LEGS/System Outputs2 ==

== system npc_controller/CONTROL/STATE-MACHINE/CPU_CONTROL_750_precharge_pfc_ok2/configGrid/FORCE_TZ/1P/LEG_A/System Outputs2 ==

== system npc_controller/CONTROL/STATE-MACHINE/CPU_CONTROL_750_precharge_pfc_ok2/configGrid/FORCE_TZ/1P/LEG_B/System Outputs2 ==

== system npc_controller/CONTROL/STATE-MACHINE/CPU_CONTROL_750_precharge_pfc_ok2/configGrid/FORCE_TZ/1P/LEG_C/System Outputs2 ==

== system npc_controller/CONTROL/STATE-MACHINE/CPU_CONTROL_750_precharge_pfc_ok2/updatePll3p/PLL/SRF_PLL/Integrator/Accumulation ==
  In1 : Inport  OutDataTypeStr=single
  Action Port : ActionPort
  Out : Outport  OutDataTypeStr=single
  wires:
  In1/1 -> Out/1

== system npc_controller/CONTROL/STATE-MACHINE/CPU_CONTROL_750_precharge_pfc_ok2/updatePll3p/PLL/SRF_PLL/Integrator/Reset Integrator ==
  Action Port : ActionPort
  Constant1 : Constant  Value=0  OutDataTypeStr=single
  Out : Outport
  wires:
  Constant1/1 -> Out/1

== system npc_controller/IDLE_AND_TIMER/codegen/CAN_Task/Rx_Handler/ProcessMB12/Debug_Cmd/Debug En//Dis ==
  Action Port : ActionPort  ActionPortLabel=if(u1 == hex2dec('0xDA'))
  Constant3 : Constant  Value=[2:2]
  Data Store Read1 : DataStoreRead  DataStoreName=u8CanDataRx12  IndexOptions=Index vector (dialog)  Indices=1  OutputSizes=1
  Debug_Dis : Subsystem  TreatAsAtomicUnit=on
  Debug_En : Subsystem  TreatAsAtomicUnit=on
  If : If  IfExpression=u1 == hex2dec('AA')  ElseIfExpressions=u1 ==hex2dec('55')
  Selector3 : Selector  IndexMode=Zero-based  InputPortWidth=8  IndexOptions=Index vector (port)  Indices=[1 3]  OutputSizes=1
  wires:
  Data Store Read1/1 -> Selector3/1
  Constant3/1 -> Selector3/2
  Selector3/1 -> If/1
  If/1 -> Debug_En/Action
  If/2 -> Debug_Dis/Action

== system npc_controller/IDLE_AND_TIMER/codegen/CAN_Task/Rx_Handler/ProcessMB12/Debug_Cmd/FUT En Dis ==
  Action Port : ActionPort  ActionPortLabel=elseif(u1 == hex2dec('0xDB'))
  Constant3 : Constant  Value=[2:2]
  Data Store Read1 : DataStoreRead  DataStoreName=u8CanDataRx12  IndexOptions=Index vector (dialog)  Indices=1  OutputSizes=1
  Disable FUT : Subsystem  TreatAsAtomicUnit=on
  Enable FUT : Subsystem  TreatAsAtomicUnit=on
  If : If  IfExpression=u1 == hex2dec('BB')  ElseIfExpressions=u1 ==hex2dec('44')
  Selector3 : Selector  IndexMode=Zero-based  InputPortWidth=8  IndexOptions=Index vector (port)  Indices=[1 3]  OutputSizes=1
  wires:
  Selector3/1 -> If/1
  Constant3/1 -> Selector3/2
  Data Store Read1/1 -> Selector3/1
  If/2 -> Disable FUT/Action
  If/1 -> Enable FUT/Action

== system npc_controller/IDLE_AND_TIMER/codegen/CAN_Task/Rx_Handler/ProcessMB12/Debug_Read/Debug_Cmd ==
  Input : Inport
  Action Port : ActionPort  ActionPortLabel=if(u1 == 1)
  Constant : Constant  OutDataTypeStr=boolean
  Data Store Write1 : DataStoreWrite  DataStoreName=b01_ReadRequest  IndexOptions=Index vector (dialog)  Indices=1  OutputSizes=1
  Data Store Write2 : DataStoreWrite  DataStoreName=u8RdReqMsgPntr  IndexOptions=Index vector (dialog)  Indices=1  OutputSizes=1
  wires:
  Constant/1 -> Data Store Write1/1
  Input/1 -> Data Store Write2/1

== system npc_controller/IDLE_AND_TIMER/codegen/CAN_Task/Tx_Handler/Run Tx Routine/TxReadRequest/ Tx FW Rev ID134 ==
  Action Port : ActionPort  ActionPortLabel=case [ 240 ]:
  CAN Pack1 : canmsglib/CAN Pack  MsgList=(none)  MsgName=CAN Msg  MsgIDType=Standard (11-bit identifier)  MsgIdentifier=0x134  MsgLength=8  Remote=off  ApplyMinMax=off  BusOutput=off  SignalInfo={}
      settings: SourceProductBaseCode=XP,ME,VN  DataFormat=raw data
  Data Store Read2 : DataStoreRead  DataStoreName=u8FwRevData  IndexOptions=Index vector (dialog)  Indices=1  OutputSizes=1
  eCAN Transmit : c280xlib/eCAN Transmit  chipFamily=C280x  useModule=eCAN_A  mailboxNo=5  messageID=hex2dec('0134')  messageType=Standard (11-bit identifier)  enableBlockingMode=off  postInterrupt=off  interruptLine=0
      settings: SourceProductBaseCode=TIC2000
  wires:
  CAN Pack1/1 -> eCAN Transmit/1
  Data Store Read2/1 -> CAN Pack1/1

== system npc_controller/IDLE_AND_TIMER/codegen/CAN_Task/Tx_Handler/Run Tx Routine/TxReadRequest/Tx Cal Data ID135 ==
  Action Port : ActionPort  ActionPortLabel=case [ 208 ]:

== system npc_controller/IDLE_AND_TIMER/codegen/CAN_Task/Tx_Handler/Run Tx Routine/TxReadRequest/Tx TxDeb Dat1 136 ==
  Action Port : ActionPort  ActionPortLabel=case [ 209 ]:
  CAN Pack1 : canmsglib/CAN Pack  MsgList=(none)  MsgName=CAN Msg  MsgIDType=Standard (11-bit identifier)  MsgIdentifier=0x136  MsgLength=8  Remote=off  ApplyMinMax=off  BusOutput=off  SignalInfo={}
      settings: SourceProductBaseCode=XP,ME,VN  DataFormat=raw data
  Constant4 : Constant  Value=0  OutDataTypeStr=uint8
  Data Store Read1 : DataStoreRead  DataStoreName=u16Debug0  IndexOptions=Index vector (dialog)  Indices=1  OutputSizes=1
  Data Store Read2 : DataStoreRead  DataStoreName=u16Debug1  IndexOptions=Index vector (dialog)  Indices=1  OutputSizes=1
  Data Store Read3 : DataStoreRead  DataStoreName=u16Debug2  IndexOptions=Index vector (dialog)  Indices=1  OutputSizes=1
  Vector Concatenate : Concatenate  NumInputs=8
  eCAN Transmit : c280xlib/eCAN Transmit  chipFamily=C280x  useModule=eCAN_A  mailboxNo=7  messageID=hex2dec('0136')  messageType=Standard (11-bit identifier)  enableBlockingMode=off  postInterrupt=off  interruptLine=0
      settings: SourceProductBaseCode=TIC2000
  u16 Data to Bytes : Subsystem
  u16 Data to Bytes1 : Subsystem
  u16 Data to Bytes2 : Subsystem
  wires:
  u16 Data to Bytes2/1(u8Lsb) -> Vector Concatenate/3
  u16 Data to Bytes/2(u8Msb) -> Vector Concatenate/2
  Data Store Read2/1 -> u16 Data to Bytes2/1(u16 Data)
  Constant4/1 -> Vector Concatenate/8, Vector Concatenate/7
  Data Store Read3/1 -> u16 Data to Bytes1/1(u16 Data)
  Vector Concatenate/1 -> CAN Pack1/1
  u16 Data to Bytes/1(u8Lsb) -> Vector Concatenate/1
  u16 Data to Bytes1/1(u8Lsb) -> Vector Concatenate/5
  Data Store Read1/1 -> u16 Data to Bytes/1(u16 Data)
  u16 Data to Bytes2/2(u8Msb) -> Vector Concatenate/4
  u16 Data to Bytes1/2(u8Msb) -> Vector Concatenate/6
  CAN Pack1/1 -> eCAN Transmit/1

== system npc_controller/IDLE_AND_TIMER/codegen/CAN_Task/Tx_Handler/Run Tx Routine/TxReadRequest/Tx TxDeb Dat2 137 ==
  Action Port : ActionPort  ActionPortLabel=case [ 210 ]:
  CAN Pack1 : canmsglib/CAN Pack  MsgList=(none)  MsgName=CAN Msg  MsgIDType=Standard (11-bit identifier)  MsgIdentifier=0x137  MsgLength=8  Remote=off  ApplyMinMax=off  BusOutput=off  SignalInfo={}
      settings: SourceProductBaseCode=XP,ME,VN  DataFormat=raw data
  Constant4 : Constant  Value=0  OutDataTypeStr=uint8
  Data Store Read1 : DataStoreRead  DataStoreName=u16Debug3  IndexOptions=Index vector (dialog)  Indices=1  OutputSizes=1
  Data Store Read2 : DataStoreRead  DataStoreName=u16Debug4  IndexOptions=Index vector (dialog)  Indices=1  OutputSizes=1
  Data Store Read3 : DataStoreRead  DataStoreName=u16Debug5  IndexOptions=Index vector (dialog)  Indices=1  OutputSizes=1
  Vector Concatenate : Concatenate  NumInputs=8
  eCAN Transmit : c280xlib/eCAN Transmit  chipFamily=C280x  useModule=eCAN_A  mailboxNo=8  messageID=hex2dec('0137')  messageType=Standard (11-bit identifier)  enableBlockingMode=off  postInterrupt=off  interruptLine=0
      settings: SourceProductBaseCode=TIC2000
  u16 Data to Bytes : Subsystem
  u16 Data to Bytes1 : Subsystem
  u16 Data to Bytes2 : Subsystem
  wires:
  u16 Data to Bytes1/2(u8Msb) -> Vector Concatenate/6
  u16 Data to Bytes2/2(u8Msb) -> Vector Concatenate/4
  u16 Data to Bytes1/1(u8Lsb) -> Vector Concatenate/5
  Data Store Read1/1 -> u16 Data to Bytes/1(u16 Data)
  Data Store Read3/1 -> u16 Data to Bytes1/1(u16 Data)
  Vector Concatenate/1 -> CAN Pack1/1
  u16 Data to Bytes/1(u8Lsb) -> Vector Concatenate/1
  CAN Pack1/1 -> eCAN Transmit/1
  Data Store Read2/1 -> u16 Data to Bytes2/1(u16 Data)
  u16 Data to Bytes/2(u8Msb) -> Vector Concatenate/2
  Constant4/1 -> Vector Concatenate/8, Vector Concatenate/7
  u16 Data to Bytes2/1(u8Lsb) -> Vector Concatenate/3

== system npc_controller/IDLE_AND_TIMER/codegen/CAN_Task/Tx_Handler/Run Tx Routine/TxStatusData/Tx Pri Status ID110 ==
  Action Port : ActionPort  ActionPortLabel=case [ 0 ]:
  CAN Pack1 : canmsglib/CAN Pack  MsgList=(none)  MsgName=CAN Msg  MsgIDType=Standard (11-bit identifier)  MsgIdentifier=0x110  MsgLength=8  Remote=off  ApplyMinMax=off  BusOutput=off  SignalInfo={}
      settings: SourceProductBaseCode=XP,ME,VN  DataFormat=raw data
  Constant1 : Constant  Value=0.1  OutDataTypeStr=single
  Constant3 : Constant  Value=0.01  OutDataTypeStr=single
  Constant4 : Constant  Value=0.1  OutDataTypeStr=single
  Data Store Read1 : DataStoreRead  DataStoreName=sPriStatus  IndexOptions=Index vector (dialog)  Indices=1  OutputSizes=1
  Data Store Read2 : DataStoreRead  DataStoreName=f32VinA  IndexOptions=Index vector (dialog)  Indices=1  OutputSizes=1
  Data Store Read3 : DataStoreRead  DataStoreName=b00_DebugEnabled  IndexOptions=Index vector (dialog)  Indices=1  OutputSizes=1
  Data Store Read4 : DataStoreRead  DataStoreName=f32IinA  IndexOptions=Index vector (dialog)  Indices=1  OutputSizes=1
  Data Store Read5 : DataStoreRead  DataStoreName=f32VpfcMid  IndexOptions=Index vector (dialog)  Indices=1  OutputSizes=1
  Float Data to Bytes : Subsystem
  Float Data to Bytes1 : Subsystem
  Float Data to Bytes2 : Subsystem
  If1 : If  IfExpression=u1 == 1
  TxReadRequest : Subsystem  TreatAsAtomicUnit=on
  Vector Concatenate : Concatenate  NumInputs=8
  eCAN Transmit : c280xlib/eCAN Transmit  chipFamily=C280x  useModule=eCAN_A  mailboxNo=0  messageID=hex2dec('0110')  messageType=Standard (11-bit identifier)  enableBlockingMode=off  postInterrupt=off  interruptLine=0
      settings: SourceProductBaseCode=TIC2000
  u16 Data to Bytes : Subsystem
  wires:
  CAN Pack1/1 -> eCAN Transmit/1
  Data Store Read3/1 -> If1/1
  If1/1 -> TxReadRequest/Action
  Data Store Read1/1 -> u16 Data to Bytes/1(u16 Data)
  u16 Data to Bytes/1(u8Lsb) -> Vector Concatenate/1
  u16 Data to Bytes/2(u8Msb) -> Vector Concatenate/2
  Vector Concatenate/1 -> CAN Pack1/1
  Constant1/1 -> Float Data to Bytes/2(Resol.)
  Data Store Read2/1 -> Float Data to Bytes/1(Float Data)
  Float Data to Bytes/1(u8Lsb) -> Vector Concatenate/3
  Float Data to Bytes/2(u8Msb) -> Vector Concatenate/4
  Data Store Read4/1 -> Float Data to Bytes1/1(Float Data)
  Constant3/1 -> Float Data to Bytes1/2(Resol.)
  Constant4/1 -> Float Data to Bytes2/2(Resol.)
  Data Store Read5/1 -> Float Data to Bytes2/1(Float Data)
  Float Data to Bytes1/1(u8Lsb) -> Vector Concatenate/5
  Float Data to Bytes1/2(u8Msb) -> Vector Concatenate/6
  Float Data to Bytes2/1(u8Lsb) -> Vector Concatenate/7
  Float Data to Bytes2/2(u8Msb) -> Vector Concatenate/8

== system npc_controller/IDLE_AND_TIMER/codegen/CAN_Task/Tx_Handler/Run Tx Routine/TxStatusData/Tx Pri1 ID130 ==
  Action Port : ActionPort  ActionPortLabel=case [ 1 ]:
  CAN Pack1 : canmsglib/CAN Pack  MsgList=(none)  MsgName=CAN Msg  MsgIDType=Standard (11-bit identifier)  MsgIdentifier=0x130  MsgLength=8  Remote=off  ApplyMinMax=off  BusOutput=off  SignalInfo={}
      settings: SourceProductBaseCode=XP,ME,VN  DataFormat=raw data
  Constant1 : Constant  Value=2  OutDataTypeStr=uint8
  Constant4 : Constant  Value=0.01  OutDataTypeStr=single
  Data Store Read1 : DataStoreRead  DataStoreName=sPriFault  IndexOptions=Index vector (dialog)  Indices=1  OutputSizes=1
  Data Store Read2 : DataStoreRead  DataStoreName=u8ThermalFlags  IndexOptions=Index vector (dialog)  Indices=1  OutputSizes=1
  Data Store Read3 : DataStoreRead  DataStoreName=u16Reserved1  IndexOptions=Index vector (dialog)  Indices=1  OutputSizes=1
  Data Store Read4 : DataStoreRead  DataStoreName=u8Reserved1  IndexOptions=Index vector (dialog)  Indices=1  OutputSizes=1
  Data Store Read5 : DataStoreRead  DataStoreName=f32Vaux  IndexOptions=Index vector (dialog)  Indices=1  OutputSizes=1
  Data Store Write1 : DataStoreWrite  DataStoreName=u8CanTxIndex  IndexOptions=Index vector (dialog)  Indices=1  OutputSizes=1
  Float Data to Bytes2 : Subsystem
  Vector Concatenate : Concatenate  NumInputs=8
  eCAN Transmit : c280xlib/eCAN Transmit  chipFamily=C280x  useModule=eCAN_A  mailboxNo=1  messageID=hex2dec('0130')  messageType=Standard (11-bit identifier)  enableBlockingMode=off  postInterrupt=off  interruptLine=0
      settings: SourceProductBaseCode=TIC2000
  u16 Data to Bytes : Subsystem
  u16 Data to Bytes1 : Subsystem
  wires:
  Constant1/1 -> Data Store Write1/1
  Data Store Read2/1 -> Vector Concatenate/3
  CAN Pack1/1 -> eCAN Transmit/1
  u16 Data to Bytes/1(u8Lsb) -> Vector Concatenate/1
  u16 Data to Bytes/2(u8Msb) -> Vector Concatenate/2
  Float Data to Bytes2/2(u8Msb) -> Vector Concatenate/8
  Constant4/1 -> Float Data to Bytes2/2(Resol.)
  Float Data to Bytes2/1(u8Lsb) -> Vector Concatenate/7
  Data Store Read5/1 -> Float Data to Bytes2/1(Float Data)
  Data Store Read1/1 -> u16 Data to Bytes/1(u16 Data)
  u16 Data to Bytes1/1(u8Lsb) -> Vector Concatenate/5
  Vector Concatenate/1 -> CAN Pack1/1
  u16 Data to Bytes1/2(u8Msb) -> Vector Concatenate/6
  Data Store Read3/1 -> u16 Data to Bytes1/1(u16 Data)
  Data Store Read4/1 -> Vector Concatenate/4
